simulink model "yarpSimTest"  (Simulink 10.0)
settings: Solver=FixedStepDiscrete  StartTime=0.0  StopTime=inf  FixedStep=0.1  RelTol=1e-3  EnableMultiTasking=on
StartFcn:
  | rx=yarpPrepare('rx',IP,yarp_port_write);
  | tx=yarpPrepare('tx',IP,yarp_port_read);
  | yarpData=zeros(2,1);
StopFcn:
  | yarpClose(rx);
  | yarpClose(tx);
  | clear rx tx yarpData;
settings Model: Creator=pattacini  LastModifiedBy=upattacini
settings DataIOCC: SignalLoggingSaveFormat=ModelDataLogs  SaveOutput=off  SignalLogging=off  DSMLogging=off  SaveTime=off
settings OptimizationCC: ExpressionDepthLimit=2147483647
settings DebuggingCC: SolverPrmCheckMsg=warning  FcnCallInpInsideContextMsg=warning  StateNameClashWarn=warning
settings GRTTargetCC: GeneratePreprocessorConditionals=Disable all
settings ConfigComp: CovExternalEMLEnable=off

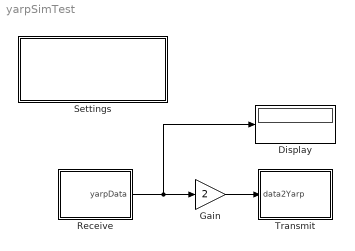
== system yarpSimTest ==
  Display : Display
  Gain : Gain  Gain=2
  Receive : MATLAB Function  TreatAsAtomicUnit=on
  Settings : Subsystem  mask{IP='10.0.75.1', yarp_port_write=10002, yarp_port_read=10003}
      mask prompts: yarp_port_write "YARP Port /write"; yarp_port_read "YARP Port /read"
      mask init:
      | assignin('base','IP',IP);
      | assignin('base','yarp_port_write',yarp_port_write);
      | assignin('base','yarp_port_read',yarp_port_read);
      mask Display:
      | IP = get_param([gcs '/Settings'],'IP');
      | yarp_port_write = str2double(get_param([gcs '/Settings'],'yarp_port_write'));
      | yarp_port_read = str2double(get_param([gcs '/Settings'],'yarp_port_read'));
      | 
      | disp(sprintf('IP = %s\nYARP Port /write = %d\nYARP Port /read = %d',...
      |              IP,yarp_port_write,yarp_port_read));
  Transmit : MATLAB Function  TreatAsAtomicUnit=on
  wires:
  Receive/1(yarpData) -> Gain/1, Display/1
  Gain/1 -> Transmit/1(data2Yarp)

== system yarpSimTest/Settings ==

== matlab function Transmit ==
  data: data2Yarp input double
function fcn(data2Yarp)

coder.extrinsic('evalin');
coder.extrinsic('num2str');

tx=evalin('base','tx');
fprintf(tx,'do');
fprintf(tx,num2str(data2Yarp'));

== matlab function Receive ==
  data: yarpData output double
function yarpData=fcn

coder.extrinsic('evalin');

yarpData=zeros(2,1);
yarpData=evalin('base','yarpData');
